simulink model "simulation_ex_1"  (R2021a)
settings: Solver=VariableStepAuto  StartTime=0.0  StopTime=10  RelTol=1e-3
settings Model: Creator=daiba  LastModifiedBy=HanO
settings SolverCC: AlgebraicLoopSolver=TrustRegion
settings DataIOCC: ReturnWorkspaceOutputs=off
settings DebuggingCC: SFMachineParentedDataDiag=warning  ArithmeticOperatorsInVariantConditions=warning
settings SFSimCC: CustomCodeUndefinedFunction=UseInterfaceOnly

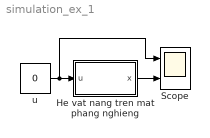
== system simulation_ex_1 ==
  He vat nang tren mat phang nghieng : Subsystem  mask{m=3, alpha=pi/6, g=9.81, x_zero=0}
      mask prompts: m "Khoi luong vat nang"; alpha "Goc mat phang nghieng"; g "Gia toc trong truong"; x_zero "Vi tri ban dau"
  Scope : Scope  NumInputPorts=2
  u : Constant  Value=0
  wires:
  u/1 -> Scope/1, He vat nang tren mat phang nghieng/1(u)
  He vat nang tren mat phang nghieng/1(x) -> Scope/2

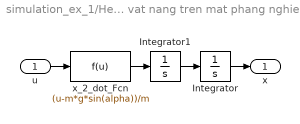
== system simulation_ex_1/He vat nang tren mat phang nghieng ==
  u : Inport
  Integrator : Integrator  InitialCondition=x_zero
  Integrator1 : Integrator
  x_2_dot_Fcn : Fcn  Expr=(u-m*g*sin(alpha))/m
  x : Outport  VectorParamsAs1DForOutWhenUnconnected=off
  wires:
  u/1 -> x_2_dot_Fcn/1
  Integrator/1 -> x/1
  x_2_dot_Fcn/1 -> Integrator1/1
  Integrator1/1 -> Integrator/1
